simulink model "penduloDifuso_2"  (R2015a)
settings: Solver=ode4  StartTime=0.0  StopTime=100.0  FixedStep=0.001  RelTol=1e-3
undefined symbols (not defined in the file): g, k, l, m, PosicionPendulo
libraries: fuzblock x1
settings Model: Creator=Benjamin Nicolas  LastModifiedBy=Benjamin Nicolas
settings SolverCC: ZeroCrossAlgorithm=Adaptive

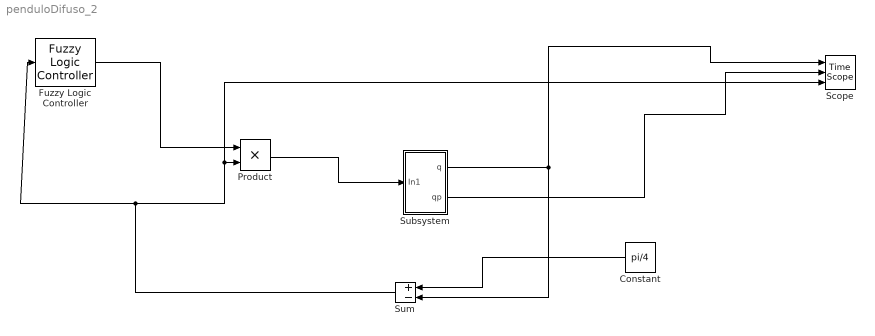
== system penduloDifuso_2 ==
  Constant : Constant  Value=pi/4
  Fuzzy Logic Controller : fuzblock/Fuzzy Logic  Controller  fis=[PosicionPendulo]
  Product : Product
  Scope : TimeScope  NumInputPorts=3
  Subsystem : Subsystem
  Sum : Sum  Inputs=+-
  wires:
  Subsystem/1("q ") -> Sum/2, Scope/1
  Subsystem/2("qp ") -> Scope/2
  Constant/1 -> Sum/1
  Fuzzy Logic Controller/1 -> Product/1
  Sum/1 -> Scope/3, Product/2, Fuzzy Logic Controller/1
  Product/1 -> Subsystem/1(In1)

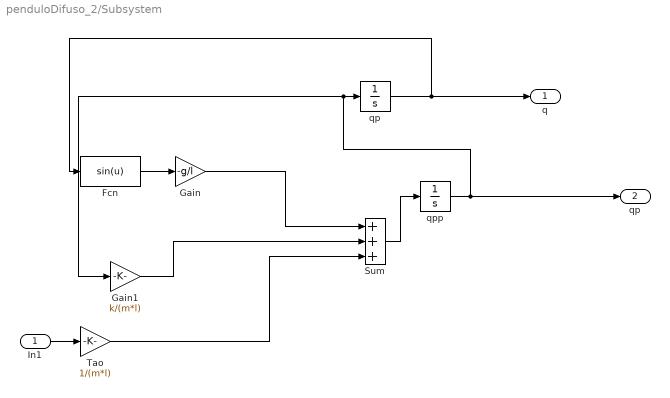
== system penduloDifuso_2/Subsystem ==
  In1 : Inport
  Fcn : Fcn  Expr=sin(u)
  Gain : Gain  Gain=-g/l
  Gain1 : Gain  Gain=k/(m*l)
  Sum : Sum  Inputs=+++
  "Tao " : Gain  Gain=1/(m*l)
  qp : Integrator
  qpp : Integrator
  "q " : Outport
  "qp " : Outport  Port=2
  wires:
  Gain1/1 -> Sum/2
  Sum/1 -> qpp/1
  Gain/1 -> Sum/1
  qp/1 -> Fcn/1, "q "/1
  Fcn/1 -> Gain/1
  qpp/1 -> "qp "/1, qp/1, Gain1/1
  In1/1 -> "Tao "/1
  "Tao "/1 -> Sum/3
